simulink model "HANcoder_E407_DYS_MP"  (R2018b)
settings: Solver=FixedStepDiscrete  StartTime=0.0  StopTime=1  FixedStep=0.01  RelTol=1e-3
PreLoadFcn:
  | librarySetup
  | eval([bdroot,'_startup']) %Calling [modelName]_startup.m
values from neighbouring files (symbols this model uses):
  basic_cycle_duration_bc0 = TM_Reset_Board   + COMP_duration    (= 212)    [HANcoder_E407_DYS_MP_startup.m]
  basic_cycle_duration_bc1 = basic_cycle_duration_bc0    (= 212)    [HANcoder_E407_DYS_MP_startup.m]
  comm_delay_estimation1 = round(comm_delay_measured1*hardware_granularity/frequency_IRQ)    [HANcoder_E407_DYS_MP_startup.m]
  comm_delay_estimation2 = round(comm_delay_measured2*hardware_granularity/frequency_IRQ)    [HANcoder_E407_DYS_MP_startup.m]
  COMM_Phase1 = Simulink.Parameter    [HANcoder_E407_DYS_MP_startup.m]
  COMM_Phase2 = Simulink.Parameter    [HANcoder_E407_DYS_MP_startup.m]
  frequency_IRQ = 500    [HANcoder_E407_DYS_MP_startup.m]
  HantuneAngleSp = Simulink.Parameter    [HANcoder_E407_DYS_MP_startup.m]
  idle_time_init = basic_cycle_duration_bc0 + basic_cycle_duration_bc1    (= 424)    [HANcoder_E407_DYS_MP_startup.m]
  matrix_rows = 2    [HANcoder_E407_DYS_MP_startup.m]
  positionD = Simulink.Parameter    [HANcoder_E407_DYS_MP_startup.m]
  positionI = Simulink.Parameter    [HANcoder_E407_DYS_MP_startup.m]
  positionP = Simulink.Parameter    [HANcoder_E407_DYS_MP_startup.m]
undefined symbols (not defined in the file or in its folder): A1, CON2, CON4, D13, Dposition, Iposition, Pposition
libraries: HANcoder_STM32_Target x33, dspswit3 x16, simulink x2, simulink_extras x2, dspstat3 x1
(part 3 of 10)

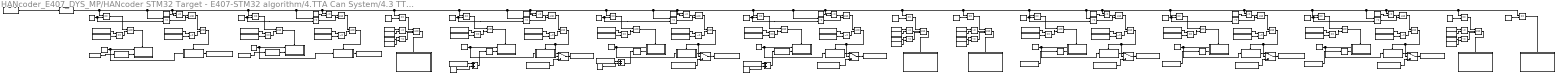
== system HANcoder_E407_DYS_MP/HANcoder STM32 Target - E407-STM32 algorithm/4.TTA Can System/4.3 TTA System/4.3.3 Matrix Cycle Manager/4.3.3.1 Controller Matrix Cycle Truck Boards 1 2 and 3/4.3.3.1.2 controller basic cycle 0.2 ==
  note: 4.3.3.1.2.1 Send Trailer Input angle 1
  note: 4.3.3.1.2.2 Receive Trailer Input angle 1
  note: 4.3.3.1.2.3 Send Trailer Input angle 2
  note: 4.3.3.1.2.4 Receive Trailer Input angle 2
  note: 4.3.3.1.2.6 Send Calc Steering Angle Board 1
  note: 4.3.3.1.2.7 Receive Calc Steering Angle Board 1
  note: 4.3.3.1.2.5 Calculate Articulation angle
  note: 4.3.3.1.2.8 Send Calc Steering Angle Board 2
  note: 4.3.3.1.2.9 Receive Calc Steering Angle Board 2
  note: 4.3.3.1.2.11 Receive Calc Steering Angle Board 3
  note: 4.3.3.1.2.10 Send Calc Steering Angle Board 3
  note: 4.3.3.1.2.12 Validate Articulation angle
  note: 4.3.3.1.2.13 Validated Angle to PWM
  note: 4.3.3.1.2.21 Check if Current id is equal to ID during initialization
  note: 4.3.3.1.2.14 Send Calc Encoder Value Board 1
  note: 4.3.3.1.2.15 Receive Calc Encoder Value Board 1
  note: 4.3.3.1.2.16 Send Calc Encoder Value Board 2
  note: 4.3.3.1.2.17 Receive Calc Encoder Value Board 2
  note: 4.3.3.1.2.19 Receive Calc Encoder Value Board 2
  note: 4.3.3.1.2.18 Send Calc Encoder Value Board 2
  note: 4.3.3.1.2.20 Check If Masters current encoder value is valid
  AND{1..6,8..16,19..27} (24 alike) : Logic  IconShape=distinctive  AllPortsSameDT=off  OutDataTypeStr=boolean
  AND{7,17..18,28} (4 alike) : Logic  Inputs=3  IconShape=distinctive  AllPortsSameDT=off  OutDataTypeStr=boolean
  Add : Sum
  Add1 : Sum
  Add2 : Sum
  Constant1 : Constant  Value=100
  Constant10 : Constant  Value=4
  Constant11 : Constant  Value=9  OutDataTypeStr=uint32
  Constant{12,17,47,50} (4 alike) : Constant  Value=2
  Constant13 : Constant  Value=95
  Constant14 : Constant  Value=94
  Constant15 : Constant  Value=99
  Constant16 : Constant  Value=8  OutDataTypeStr=uint32
  Constant18 : Constant  Value=105
  Constant19 : Constant  Value=109
  Constant{2,20..21,30,32,41,44,55} (8 alike) : Constant
  Constant22 : Constant  Value=5
  Constant23 : Constant  Value=4
  Constant{5,24..25,31,33,51,53,56} (8 alike) : Constant  Value=3
  Constant26 : Constant  Value=6  OutDataTypeStr=uint32
  Constant27 : Constant  Value=115
  Constant28 : Constant  Value=119
  Constant29 : Constant  Value=120
  Constant3 : Constant  Value=10  OutDataTypeStr=uint32
  Constant34 : Constant  Value=121
  Constant35 : Constant  Value=5  OutDataTypeStr=uint32
  Constant{8,36,38..39} (4 alike) : Constant  Value=90
  Constant37 : Constant  Value=138
  Constant4 : Constant  Value=7  OutDataTypeStr=uint32
  Constant40 : Constant  Value=122
  Constant42 : Constant  Value=3  OutDataTypeStr=uint32
  Constant43 : Constant  Value=126
  Constant45 : Constant  Value=4  OutDataTypeStr=uint32
  Constant46 : Constant  Value=127
  Constant48 : Constant  Value=132
  Constant49 : Constant  Value=131
  Constant52 : Constant  Value=136
  Constant54 : Constant  Value=137
  Constant6 : Constant  Value=110
  Constant7 : Constant  Value=114
  Constant9 : Constant  Value=5
  Data Store Read{,1..3,5..7,9,13..14,16..21,26,28,30,32,34,36..38} (24 alike) : DataStoreRead  DataStoreName=Board_ID
  Data Store Read10 : DataStoreRead  DataStoreName=Votes_Angle  DataStoreElements=Votes_Angle.First_Board
  Data Store Read11 : DataStoreRead  DataStoreName=Votes_Angle  DataStoreElements=Votes_Angle.Second_Board
  Data Store Read12 : DataStoreRead  DataStoreName=CalcSteeringAngle
  Data Store Read15 : DataStoreRead  DataStoreName=CalcSteeringAngle
  Data Store Read22 : DataStoreRead  DataStoreName=Votes_Angle  DataStoreElements=Votes_Angle.Third_Board
  Data Store Read23 : DataStoreRead  DataStoreName=PotAngle
  Data Store Read24 : DataStoreRead  DataStoreName=PotAngle
  Data Store Read25 : DataStoreRead  DataStoreName=EncoderValue
  Data Store Read27 : DataStoreRead  DataStoreName=Votes_Encoder  DataStoreElements=Votes_Encoder.First_Board
  Data Store Read29 : DataStoreRead  DataStoreName=EncoderValue
  Data Store Read31 : DataStoreRead  DataStoreName=Votes_Encoder  DataStoreElements=Votes_Encoder.Second_Board
  Data Store Read33 : DataStoreRead  DataStoreName=EncoderValue
  Data Store Read35 : DataStoreRead  DataStoreName=Votes_Encoder  DataStoreElements=Votes_Encoder.Third_Board
  Data Store Read4 : DataStoreRead  DataStoreName=CalcSteeringAngle
  Data Store Read8 : DataStoreRead  DataStoreName=Local_Ticks
  Data Store Write : DataStoreWrite  DataStoreName=InputAngle1
  Data Store Write1 : DataStoreWrite  DataStoreName=InputAngle2
  Data Store Write2 : DataStoreWrite  DataStoreName=Votes_Angle  DataStoreElements=Votes_Angle.First_Board
  Data Store Write3 : DataStoreWrite  DataStoreName=Votes_Angle  DataStoreElements=Votes_Angle.Second_Board
  Data Store Write4 : DataStoreWrite  DataStoreName=Votes_Angle  DataStoreElements=Votes_Angle.Third_Board
  Data Store Write6 : DataStoreWrite  DataStoreName=Votes_Encoder  DataStoreElements=Votes_Encoder.First_Board
  Data Store Write7 : DataStoreWrite  DataStoreName=Votes_Encoder  DataStoreElements=Votes_Encoder.Second_Board
  Data Store Write8 : DataStoreWrite  DataStoreName=Votes_Encoder  DataStoreElements=Votes_Encoder.Third_Board
  Data Type Conversion{1..2,4..9} (8 alike) : DataTypeConversion  OutDataTypeStr=uint8
  Data Type Conversion3 : DataTypeConversion  OutDataTypeStr=double
  Equal{1,13,15,23} (4 alike) : RelationalOperator  OutDataTypeStr=boolean  RndMeth=Simplest
  Equal{5..7,10..11,17,19,21} (8 alike) : RelationalOperator  Operator===  OutDataTypeStr=boolean  RndMeth=Simplest
  Equal{2..4,9,12,18,20,22} (8 alike) : RelationalOperator  Operator=~=  OutDataTypeStr=boolean  RndMeth=Simplest
  Equal{8,14,16,24} (4 alike) : RelationalOperator  Operator=<=  OutDataTypeStr=boolean  RndMeth=Simplest
  GreaterThanOrEqual{1..2,4,6,10,15,17..20,23,26,29} (13 alike) : RelationalOperator  Operator===  OutDataTypeStr=boolean  RndMeth=Simplest
  GreaterThanOrEqual{3,5,7,11,16,21,24,27} (8 alike) : RelationalOperator  OutDataTypeStr=boolean  RndMeth=Simplest
  GreaterThanOrEqual{8..9,12..14,22,25,28} (8 alike) : RelationalOperator  Operator=<=  OutDataTypeStr=boolean  RndMeth=Simplest
  If Action Subsystem : Subsystem  TreatAsAtomicUnit=on
  If Action Subsystem1 : Subsystem  TreatAsAtomicUnit=on
  If Action Subsystem2 : Subsystem  TreatAsAtomicUnit=on
  If Action Subsystem3 : Subsystem  TreatAsAtomicUnit=on
  If Action Subsystem4 : Subsystem  TreatAsAtomicUnit=on
  Receive Trailer 1 board 4 input angel : Subsystem
  Receive Trailer 2 board 5 input angel : Subsystem
  Receive Truck 1 Board 1 Calc Steering Angle : Subsystem
  Receive Truck 1 Board 1 Calc Steering Angle1 : Subsystem
  Receive Truck 1 Board 1 Calc Steering Angle2 : Subsystem
  Receive Truck 1 Board 1 Calc Steering Angle3 : Subsystem
  Receive Truck 2 Board 2 Calc Steering Angle : Subsystem
  Receive Truck 3 Board 3 Calc Steering Angle : Subsystem
  Send can message : Subsystem  TreatAsAtomicUnit=on
  Send can message1 : Subsystem  TreatAsAtomicUnit=on
  Send can message2 : Subsystem  TreatAsAtomicUnit=on
  Send can message3 : Subsystem  TreatAsAtomicUnit=on
  Send can message4 : Subsystem  TreatAsAtomicUnit=on
  Send can message5 : Subsystem  TreatAsAtomicUnit=on
  Send can message6 : Subsystem  TreatAsAtomicUnit=on
  Send can message7 : Subsystem  TreatAsAtomicUnit=on
  Switch{,1..5} (6 alike) : Switch  Criteria=u2 > Threshold
  wires:
  Data Store Read8/1 -> Data Type Conversion3/1
  Constant8/1 -> GreaterThanOrEqual5/2, GreaterThanOrEqual4/2
  Equal2/1 -> AND9/2
  Data Store Read/1 -> Equal2/1
  Constant10/1 -> Equal2/2
  AND9/1 -> Receive Trailer 1 board 4 input angel/Enable
  Constant3/1 -> Receive Trailer 1 board 4 input angel/1(Input), Send can message/1(Can_ID)
  AND6/1 -> Receive Trailer 2 board 5 input angel/Enable
  Constant13/1 -> GreaterThanOrEqual7/2, GreaterThanOrEqual6/2
  Data Store Read2/1 -> Equal3/1
  Equal3/1 -> AND6/2
  Constant9/1 -> Equal3/2
  Constant11/1 -> Receive Trailer 2 board 5 input angel/1(Input), Send can message1/1(Can_ID)
  Constant14/1 -> GreaterThanOrEqual8/2
  GreaterThanOrEqual8/1 -> AND3/1
  GreaterThanOrEqual5/1 -> AND3/2
  AND3/1 -> AND9/1
  Receive Trailer 1 board 4 input angel/1(Angle) -> Data Store Write/1
  Constant15/1 -> GreaterThanOrEqual9/2
  GreaterThanOrEqual9/1 -> AND4/1
  GreaterThanOrEqual7/1 -> AND4/2
  AND4/1 -> AND6/1
  Receive Trailer 2 board 5 input angel/1(Angle) -> Data Store Write1/1
  Constant18/1 -> GreaterThanOrEqual11/2, GreaterThanOrEqual10/2
  GreaterThanOrEqual11/1 -> AND5/2
  AND2/1 -> Switch/2, Receive Truck 1 Board 1 Calc Steering Angle/Enable
  Constant16/1 -> Receive Truck 1 Board 1 Calc Steering Angle/1(Input), Send can message2/1(Can_ID)
  Constant20/1 -> Equal4/2
  Equal4/1 -> AND2/2
  AND5/1 -> AND2/1
  GreaterThanOrEqual12/1 -> AND5/1
  Data Store Read5/1 -> Equal4/1
  Constant19/1 -> GreaterThanOrEqual12/2
  Equal5/1 -> AND1/2
  Constant21/1 -> Equal5/2
  Data Store Read6/1 -> Equal5/1
  AND1/1 -> Send can message2/Enable
  GreaterThanOrEqual10/1 -> AND1/1
  Equal6/1 -> AND8/2
  Constant22/1 -> Equal6/2
  Data Store Read7/1 -> Equal6/1
  GreaterThanOrEqual6/1 -> AND8/1
  AND8/1 -> Send can message1/Enable
  GreaterThanOrEqual4/1 -> AND10/1
  Data Store Read9/1 -> Equal7/1
  Constant23/1 -> Equal7/2
  Equal7/1 -> AND10/2
  AND10/1 -> Send can message/Enable
  Constant1/1 -> GreaterThanOrEqual1/2
  GreaterThanOrEqual1/1 -> AND7/1
  AND7/1 -> If Action Subsystem/Enable
  Data Store Read1/1 -> Equal1/1
  Constant2/1 -> Equal1/2
  Equal1/1 -> AND7/2
  Constant5/1 -> Equal8/2
  Data Store Read3/1 -> Equal8/1
  Equal8/1 -> AND7/3
  GreaterThanOrEqual3/1 -> AND13/2
  Data Store Read14/1 -> Equal10/1
  Constant7/1 -> GreaterThanOrEqual13/2
  GreaterThanOrEqual13/1 -> AND13/1
  Constant4/1 -> Receive Truck 2 Board 2 Calc Steering Angle/1(Input), Send can message3/1(Can_ID)
  Constant6/1 -> GreaterThanOrEqual3/2, GreaterThanOrEqual2/2
  Constant17/1 -> Equal10/2
  GreaterThanOrEqual2/1 -> AND11/1
  Equal10/1 -> AND11/2
  AND11/1 -> Send can message3/Enable
  Data Store Read13/1 -> Equal9/1
  Constant12/1 -> Equal9/2
  AND13/1 -> AND12/1
  Equal9/1 -> AND12/2
  GreaterThanOrEqual14/1 -> AND16/1
  Data Store Read17/1 -> Equal11/1
  GreaterThanOrEqual16/1 -> AND16/2
  Constant28/1 -> GreaterThanOrEqual14/2
  Equal12/1 -> AND15/2
  Equal11/1 -> AND14/2
  GreaterThanOrEqual15/1 -> AND14/1
  AND16/1 -> AND15/1
  Data Store Read16/1 -> Equal12/1
  AND14/1 -> Send can message4/Enable
  Constant27/1 -> GreaterThanOrEqual16/2, GreaterThanOrEqual15/2
  Constant25/1 -> Equal11/2
  Constant26/1 -> Receive Truck 3 Board 3 Calc Steering Angle/1(Input), Send can message4/1(Can_ID)
  Constant24/1 -> Equal12/2
  Data Store Read19/1 -> Equal14/1
  GreaterThanOrEqual17/1 -> AND17/1
  AND17/1 -> If Action Subsystem1/Enable
  Constant29/1 -> GreaterThanOrEqual17/2
  Constant30/1 -> Equal13/2
  Constant31/1 -> Equal14/2
  Data Store Read18/1 -> Equal13/1
  Equal14/1 -> AND17/3
  Equal13/1 -> AND17/2
  Data Store Read20/1 -> Equal15/1
  Equal16/1 -> AND18/3
  Equal15/1 -> AND18/2
  Constant32/1 -> Equal15/2
  Constant33/1 -> Equal16/2
  GreaterThanOrEqual18/1 -> AND18/1
  Data Store Read21/1 -> Equal16/1
  Constant34/1 -> GreaterThanOrEqual18/2
  AND18/1 -> If Action Subsystem2/Enable
  GreaterThanOrEqual19/1 -> If Action Subsystem3/Enable
  Constant37/1 -> GreaterThanOrEqual19/2
  Data Store Read24/1 -> Data Type Conversion2/1
  Data Type Conversion2/1 -> Send can message1/2(Can_Data)
  Data Type Conversion1/1 -> Send can message/2(Can_Data)
  Data Store Read23/1 -> Data Type Conversion1/1
  Data Type Conversion4/1 -> Send can message2/2(Can_Data)
  Data Type Conversion5/1 -> Send can message3/2(Can_Data)
  Data Type Conversion6/1 -> Send can message4/2(Can_Data)
  Data Store Read12/1 -> Add/1
  Constant36/1 -> Add/2
  Add/1 -> Data Type Conversion5/1
  Constant38/1 -> Add1/2
  Data Store Read15/1 -> Add1/1
  Add1/1 -> Data Type Conversion6/1
  Constant39/1 -> Add2/2
  Add2/1 -> Data Type Conversion4/1  "testtest"
  Data Store Read4/1 -> Add2/1  "test1"
  Switch/1 -> Data Store Write2/1
  Receive Truck 1 Board 1 Calc Steering Angle/1(Angle) -> Switch/1
  Data Store Read10/1 -> Switch/3
  AND12/1 -> Switch1/2, Receive Truck 2 Board 2 Calc Steering Angle/Enable
  Data Store Read11/1 -> Switch1/3
  Receive Truck 2 Board 2 Calc Steering Angle/1(Angle) -> Switch1/1
  Switch1/1 -> Data Store Write3/1
  Switch2/1 -> Data Store Write4/1
  AND15/1 -> Switch2/2, Receive Truck 3 Board 3 Calc Steering Angle/Enable
  Data Store Read22/1 -> Switch2/3
  Receive Truck 3 Board 3 Calc Steering Angle/1(Angle) -> Switch2/1
  Constant41/1 -> Equal17/2
  Data Store Read25/1 -> Data Type Conversion7/1
  Data Type Conversion7/1 -> Send can message5/2(Can_Data)
  Constant40/1 -> GreaterThanOrEqual21/2, GreaterThanOrEqual20/2
  Data Store Read26/1 -> Equal17/1
  Equal17/1 -> AND19/2
  GreaterThanOrEqual20/1 -> AND19/1
  AND19/1 -> Send can message5/Enable
  GreaterThanOrEqual21/1 -> AND21/2
  Constant43/1 -> GreaterThanOrEqual22/2
  Data Store Read28/1 -> Equal18/1
  AND21/1 -> AND20/1
  GreaterThanOrEqual22/1 -> AND21/1
  Constant35/1 -> Receive Truck 1 Board 1 Calc Steering Angle1/1(Input), Send can message5/1(Can_ID)
  Constant44/1 -> Equal18/2
  Receive Truck 1 Board 1 Calc Steering Angle1/1(Angle) -> Switch3/1
  AND20/1 -> Switch3/2, Receive Truck 1 Board 1 Calc Steering Angle1/Enable
  Data Store Read27/1 -> Switch3/3
  Switch3/1 -> Data Store Write6/1
  Equal18/1 -> AND20/2
  Switch4/1 -> Data Store Write7/1
  Data Store Read29/1 -> Data Type Conversion8/1
  AND23/1 -> Switch4/2, Receive Truck 1 Board 1 Calc Steering Angle2/Enable
  Equal20/1 -> AND23/2
  Receive Truck 1 Board 1 Calc Steering Angle2/1(Angle) -> Switch4/1
  Data Store Read31/1 -> Switch4/3
  GreaterThanOrEqual25/1 -> AND24/1
  Data Store Read32/1 -> Equal20/1
  AND24/1 -> AND23/1
  GreaterThanOrEqual24/1 -> AND24/2
  Constant50/1 -> Equal20/2
  AND22/1 -> Send can message6/Enable
  Constant49/1 -> GreaterThanOrEqual25/2
  Constant45/1 -> Receive Truck 1 Board 1 Calc Steering Angle2/1(Input), Send can message6/1(Can_ID)
  Equal19/1 -> AND22/2
  Data Store Read30/1 -> Equal19/1
  Data Type Conversion8/1 -> Send can message6/2(Can_Data)
  Constant46/1 -> GreaterThanOrEqual24/2, GreaterThanOrEqual23/2
  GreaterThanOrEqual23/1 -> AND22/1
  Constant47/1 -> Equal19/2
  Constant51/1 -> Equal21/2
  Constant52/1 -> GreaterThanOrEqual28/2
  AND25/1 -> Send can message7/Enable
  Constant53/1 -> Equal22/2
  GreaterThanOrEqual27/1 -> AND27/2
  AND27/1 -> AND26/1
  GreaterThanOrEqual28/1 -> AND27/1
  Data Store Read36/1 -> Equal22/1
  Receive Truck 1 Board 1 Calc Steering Angle3/1(Angle) -> Switch5/1
  Equal22/1 -> AND26/2
  AND26/1 -> Switch5/2, Receive Truck 1 Board 1 Calc Steering Angle3/Enable
  Switch5/1 -> Data Store Write8/1
  Data Store Read35/1 -> Switch5/3
  Constant48/1 -> GreaterThanOrEqual27/2, GreaterThanOrEqual26/2
  Data Store Read34/1 -> Equal21/1
  Data Type Conversion9/1 -> Send can message7/2(Can_Data)
  Equal21/1 -> AND25/2
  Constant42/1 -> Receive Truck 1 Board 1 Calc Steering Angle3/1(Input), Send can message7/1(Can_ID)
  Data Store Read33/1 -> Data Type Conversion9/1
  GreaterThanOrEqual26/1 -> AND25/1
  Data Type Conversion3/1 -> GreaterThanOrEqual8/1, GreaterThanOrEqual11/1, GreaterThanOrEqual3/1, GreaterThanOrEqual21/1, GreaterThanOrEqual22/1, GreaterThanOrEqual23/1, GreaterThanOrEqual25/1, GreaterThanOrEqual26/1, GreaterThanOrEqual27/1, GreaterThanOrEqual28/1, GreaterThanOrEqual29/1, GreaterThanOrEqual19/1, GreaterThanOrEqual20/1, GreaterThanOrEqual18/1, GreaterThanOrEqual17/1, GreaterThanOrEqual14/1, GreaterThanOrEqual16/1, GreaterThanOrEqual15/1, GreaterThanOrEqual13/1, GreaterThanOrEqual2/1, GreaterThanOrEqual12/1, GreaterThanOrEqual10/1, GreaterThanOrEqual1/1, GreaterThanOrEqual9/1, GreaterThanOrEqual7/1, GreaterThanOrEqual6/1, GreaterThanOrEqual5/1, GreaterThanOrEqual4/1
  Constant56/1 -> Equal24/2
  AND28/1 -> If Action Subsystem4/Enable
  Data Store Read37/1 -> Equal23/1
  Constant55/1 -> Equal23/2
  Equal24/1 -> AND28/3
  Equal23/1 -> AND28/2
  GreaterThanOrEqual29/1 -> AND28/1
  Data Store Read38/1 -> Equal24/1
  Constant54/1 -> GreaterThanOrEqual29/2

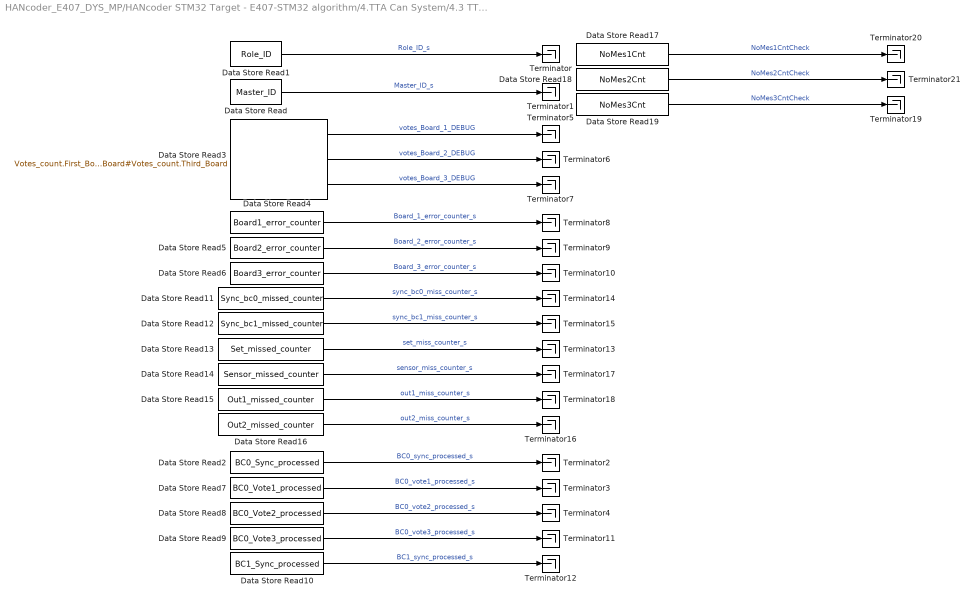
== system HANcoder_E407_DYS_MP/HANcoder STM32 Target - E407-STM32 algorithm/4.TTA Can System/4.3 TTA System/4.3.3 Matrix Cycle Manager/4.3.3.1 Controller Matrix Cycle Truck Boards 1 2 and 3/Matrix_Cycle_Observation_DEBUG ==
  Data Store Read : DataStoreRead  DataStoreName=Master_ID
  Data Store Read1 : DataStoreRead  DataStoreName=Role_ID
  Data Store Read10 : DataStoreRead  DataStoreName=BC1_Sync_processed
  Data Store Read11 : DataStoreRead  DataStoreName=Sync_bc0_missed_counter
  Data Store Read12 : DataStoreRead  DataStoreName=Sync_bc1_missed_counter
  Data Store Read13 : DataStoreRead  DataStoreName=Set_missed_counter
  Data Store Read14 : DataStoreRead  DataStoreName=Sensor_missed_counter
  Data Store Read15 : DataStoreRead  DataStoreName=Out1_missed_counter
  Data Store Read16 : DataStoreRead  DataStoreName=Out2_missed_counter
  Data Store Read17 : DataStoreRead  DataStoreName=NoMes1Cnt
  Data Store Read18 : DataStoreRead  DataStoreName=NoMes2Cnt
  Data Store Read19 : DataStoreRead  DataStoreName=NoMes3Cnt
  Data Store Read2 : DataStoreRead  DataStoreName=BC0_Sync_processed
  Data Store Read3 : DataStoreRead  DataStoreName=Votes_count  DataStoreElements=Votes_count.First_Board#Votes_count.Second_Board#Votes_count.Third_Board
  Data Store Read4 : DataStoreRead  DataStoreName=Board1_error_counter
  Data Store Read5 : DataStoreRead  DataStoreName=Board2_error_counter
  Data Store Read6 : DataStoreRead  DataStoreName=Board3_error_counter
  Data Store Read7 : DataStoreRead  DataStoreName=BC0_Vote1_processed
  Data Store Read8 : DataStoreRead  DataStoreName=BC0_Vote2_processed
  Data Store Read9 : DataStoreRead  DataStoreName=BC0_Vote3_processed
  Terminator{,1..21} (22 alike) : Terminator
  wires:
  Data Store Read/1 -> Terminator1/1  "Master_ID_s"
  Data Store Read3/1 -> Terminator5/1  "votes_Board_1_DEBUG"
  Data Store Read3/2 -> Terminator6/1  "votes_Board_2_DEBUG"
  Data Store Read3/3 -> Terminator7/1  "votes_Board_3_DEBUG"
  Data Store Read4/1 -> Terminator8/1  "Board_1_error_counter_s"
  Data Store Read5/1 -> Terminator9/1  "Board_2_error_counter_s"
  Data Store Read6/1 -> Terminator10/1  "Board_3_error_counter_s"
  Data Store Read2/1 -> Terminator2/1  "BC0_sync_processed_s"
  Data Store Read7/1 -> Terminator3/1  "BC0_vote1_processed_s"
  Data Store Read8/1 -> Terminator4/1  "BC0_vote2_processed_s"
  Data Store Read9/1 -> Terminator11/1  "BC0_vote3_processed_s"
  Data Store Read10/1 -> Terminator12/1  "BC1_sync_processed_s"
  Data Store Read1/1 -> Terminator/1  "Role_ID_s"
  Data Store Read11/1 -> Terminator14/1  "sync_bc0_miss_counter_s"
  Data Store Read12/1 -> Terminator15/1  "sync_bc1_miss_counter_s"
  Data Store Read13/1 -> Terminator13/1  "set_miss_counter_s"
  Data Store Read14/1 -> Terminator17/1  "sensor_miss_counter_s"
  Data Store Read15/1 -> Terminator18/1  "out1_miss_counter_s"
  Data Store Read16/1 -> Terminator16/1  "out2_miss_counter_s"
  Data Store Read17/1 -> Terminator20/1  "NoMes1CntCheck"
  Data Store Read18/1 -> Terminator21/1  "NoMes2CntCheck"
  Data Store Read19/1 -> Terminator19/1  "NoMes3CntCheck"

== system HANcoder_E407_DYS_MP/HANcoder STM32 Target - E407-STM32 algorithm/4.TTA Can System/4.3 TTA System/4.3.3 Matrix Cycle Manager/4.3.3.1 Controller Matrix Cycle Truck Boards 1 2 and 3/msg_count_DEBUG observer ==
  Data Store Read24 : DataStoreRead  DataStoreName=msg_count_DEBUG
  Terminator : Terminator
  wires:
  Data Store Read24/1 -> Terminator/1  "msg_count_DEBUG_s"

== system HANcoder_E407_DYS_MP/HANcoder STM32 Target - E407-STM32 algorithm/4.TTA Can System/4.3 TTA System/4.3.3 Matrix Cycle Manager/4.3.3.2 Controller Matrix Cycle_Board 4 and 5/controller basic cycle 0 ==
  note: Receving Time Window
  note: Receving Time Window
  AND : Logic  IconShape=distinctive  AllPortsSameDT=off  OutDataTypeStr=boolean
  AND1 : Logic  IconShape=distinctive  AllPortsSameDT=off  OutDataTypeStr=boolean
  AND2 : Logic  IconShape=distinctive  AllPortsSameDT=off  OutDataTypeStr=boolean
  Constant : Constant  Value=25
  Constant5 : Constant  Value=5
  Constant6 : Constant  Value=60
  Constant7 : Constant  Value=61
  Counter1 : dspswit3/Counter  Direction=Up  CountEvent=Rising edge  CounterSize=User defined  MaxCount=255  InitialCount=0  Output=Count and Hit  HitValue=32  ResetInput=on  SamplesPerFrame=1  Ts=1  CntDtype=double  HitDtype=Logical
  Counter3 : dspswit3/Counter  Direction=Up  CountEvent=Rising edge  CounterSize=User defined  MaxCount=255  InitialCount=0  Output=Count and Hit  HitValue=32  ResetInput=on  SamplesPerFrame=1  Ts=1  CntDtype=double  HitDtype=Logical
  Data Store Memory3 : DataStoreMemory  DataStoreName=SyncMesRec  ReadBeforeWriteMsg=warning  WriteAfterWriteMsg=warning  WriteAfterReadMsg=warning  ShowAdditionalParam=off  OutMin=0  OutMax=255  OutDataTypeStr=uint8
  Data Store Read3 : DataStoreRead  Priority=10  DataStoreName=Role_ID
  Data Store Read4 : DataStoreRead  DataStoreName=SyncMesRec
  Data Store Read8 : DataStoreRead  DataStoreName=Local_Ticks
  Data Type Conversion3 : DataTypeConversion  OutDataTypeStr=double
  Desync calculation : Subsystem  Priority=10
  GreaterThanOrEqual : RelationalOperator  Operator=>  OutDataTypeStr=boolean  RndMeth=Simplest
  GreaterThanOrEqual1 : RelationalOperator  Operator=<=  OutDataTypeStr=boolean  RndMeth=Simplest
  GreaterThanOrEqual2 : RelationalOperator  Operator=>  OutDataTypeStr=boolean  RndMeth=Simplest
  GreaterThanOrEqual3 : RelationalOperator  Operator=<=  OutDataTypeStr=boolean  RndMeth=Simplest
  If Action Subsystem : Subsystem  TreatAsAtomicUnit=on
  OR : Logic  Operator=OR  IconShape=distinctive  AllPortsSameDT=off  OutDataTypeStr=boolean
  "Receive Timer can master message " : Subsystem
  Terminator1 : Terminator
  Terminator4 : Terminator
  wires:
  Data Store Read8/1 -> Data Type Conversion3/1
  Data Type Conversion3/1 -> GreaterThanOrEqual/1, GreaterThanOrEqual1/1, GreaterThanOrEqual2/1, GreaterThanOrEqual3/1
  Data Store Read3/1 -> "Receive Timer can master message "/1(Sender Id)
  Constant/1 -> Desync calculation/1(TM_COMM)
  "Receive Timer can master message "/2(Can1Rec) -> OR/1, Desync calculation/2(New_msg_CAN1)
  "Receive Timer can master message "/4(Can2Rec) -> OR/2
  OR/1 -> Counter1/1, Desync calculation/Enable
  Constant5/1 -> GreaterThanOrEqual/2
  GreaterThanOrEqual/1 -> AND/2
  Constant6/1 -> GreaterThanOrEqual2/2, GreaterThanOrEqual1/2
  GreaterThanOrEqual1/1 -> AND/1
  Constant7/1 -> GreaterThanOrEqual3/2
  GreaterThanOrEqual3/1 -> AND1/1
  GreaterThanOrEqual2/1 -> AND1/2
  AND2/1 -> If Action Subsystem/Enable
  Counter1/1 -> Terminator1/1
  Counter3/1 -> Terminator4/1
  AND/1 -> Counter3/1, "Receive Timer can master message "/Enable
  AND1/1 -> AND2/1
  Data Store Read4/1 -> AND2/2

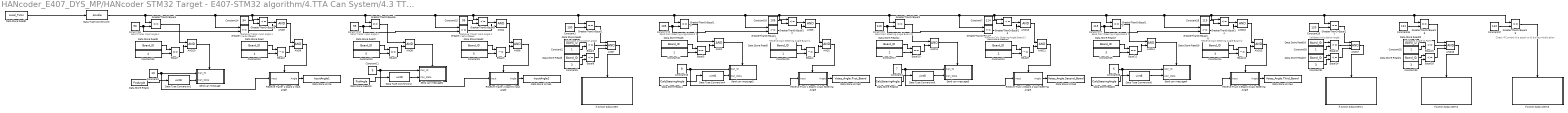
== system HANcoder_E407_DYS_MP/HANcoder STM32 Target - E407-STM32 algorithm/4.TTA Can System/4.3 TTA System/4.3.3 Matrix Cycle Manager/4.3.3.2 Controller Matrix Cycle_Board 4 and 5/controller basic cycle 0.2 ==
  note: Send Trailer Input angle 1
  note: Receive Trailer Input angle 1
  note: Send Trailer Input angle 2
  note: Receive Trailer Input angle 2
  note: Send Calc Steering Angle Board 1
  note: Receive Calc Steering Angle Board 1
  note: Calculate Articulation angle
  note: Send Calc Steering Angle Board 2
  note: Receive Calc Steering Angle Board 2
  note: Receive Calc Steering Angle Board 2
  note: Send Calc Steering Angle Board 2
  note: Validate Articulation angle
  note: Validated Angle to PWM
  note: Check if Current id is equal to ID during initialization
  AND{1..6,8..16} (15 alike) : Logic  IconShape=distinctive  AllPortsSameDT=off  OutDataTypeStr=boolean
  AND17 : Logic  Inputs=3  IconShape=distinctive  AllPortsSameDT=off  OutDataTypeStr=boolean
  AND18 : Logic  Inputs=3  IconShape=distinctive  AllPortsSameDT=off  OutDataTypeStr=boolean
  AND7 : Logic  Inputs=3  IconShape=distinctive  AllPortsSameDT=off  OutDataTypeStr=boolean
  Constant1 : Constant  Value=100
  Constant10 : Constant  Value=4
  Constant11 : Constant  Value=9  OutDataTypeStr=uint32
  Constant12 : Constant  Value=2
  Constant13 : Constant  Value=95
  Constant14 : Constant  Value=94
  Constant15 : Constant  Value=99
  Constant16 : Constant  Value=8  OutDataTypeStr=uint32
  Constant17 : Constant  Value=2
  Constant18 : Constant  Value=105
  Constant19 : Constant  Value=109
  Constant{2,20..21,30,32} (5 alike) : Constant
  Constant22 : Constant  Value=5
  Constant23 : Constant  Value=4
  Constant{5,24..25,31,33} (5 alike) : Constant  Value=3
  Constant26 : Constant  Value=6  OutDataTypeStr=uint32
  Constant27 : Constant  Value=115
  Constant28 : Constant  Value=119
  Constant29 : Constant  Value=120
  Constant3 : Constant  Value=10  OutDataTypeStr=uint32
  Constant34 : Constant  Value=121
  Constant37 : Constant  Value=122
  Constant4 : Constant  Value=7  OutDataTypeStr=uint32
  Constant6 : Constant  Value=110
  Constant7 : Constant  Value=114
  Constant8 : Constant  Value=90
  Constant9 : Constant  Value=5
  Data Store Read{,1..3,5..7,9,13..14,16..21} (16 alike) : DataStoreRead  DataStoreName=Board_ID
  Data Store Read10 : DataStoreRead  DataStoreName=PotAngle
  Data Store Read11 : DataStoreRead  DataStoreName=CalcSteeringAngle
  Data Store Read12 : DataStoreRead  DataStoreName=CalcSteeringAngle
  Data Store Read15 : DataStoreRead  DataStoreName=CalcSteeringAngle
  Data Store Read4 : DataStoreRead  DataStoreName=PotAngle
  Data Store Read8 : DataStoreRead  DataStoreName=Local_Ticks
  Data Store Write : DataStoreWrite  DataStoreName=InputAngle1
  Data Store Write1 : DataStoreWrite  DataStoreName=InputAngle2
  Data Store Write2 : DataStoreWrite  DataStoreName=Votes_Angle  DataStoreElements=Votes_Angle.First_Board
  Data Store Write3 : DataStoreWrite  DataStoreName=Votes_Angle  DataStoreElements=Votes_Angle.Second_Board
  Data Store Write4 : DataStoreWrite  DataStoreName=Votes_Angle  DataStoreElements=Votes_Angle.Third_Board
  Data Type Conversion{1..2,4..6} (5 alike) : DataTypeConversion  OutDataTypeStr=uint8
  Data Type Conversion3 : DataTypeConversion  OutDataTypeStr=double
  Equal1 : RelationalOperator  OutDataTypeStr=boolean  RndMeth=Simplest
  Equal{5..7,10..11} (5 alike) : RelationalOperator  Operator===  OutDataTypeStr=boolean  RndMeth=Simplest
  Equal{2..4,9,12} (5 alike) : RelationalOperator  Operator=~=  OutDataTypeStr=boolean  RndMeth=Simplest
  Equal13 : RelationalOperator  OutDataTypeStr=boolean  RndMeth=Simplest
  Equal14 : RelationalOperator  Operator=<=  OutDataTypeStr=boolean  RndMeth=Simplest
  Equal15 : RelationalOperator  OutDataTypeStr=boolean  RndMeth=Simplest
  Equal16 : RelationalOperator  Operator=<=  OutDataTypeStr=boolean  RndMeth=Simplest
  Equal8 : RelationalOperator  Operator=<=  OutDataTypeStr=boolean  RndMeth=Simplest
  GreaterThanOrEqual{1..2,4,6,10,15,17..19} (9 alike) : RelationalOperator  Operator===  OutDataTypeStr=boolean  RndMeth=Simplest
  GreaterThanOrEqual{3,5,7,11,16} (5 alike) : RelationalOperator  OutDataTypeStr=boolean  RndMeth=Simplest
  GreaterThanOrEqual{8..9,12..14} (5 alike) : RelationalOperator  Operator=<=  OutDataTypeStr=boolean  RndMeth=Simplest
  If Action Subsystem : Subsystem  TreatAsAtomicUnit=on
  If Action Subsystem1 : Subsystem  TreatAsAtomicUnit=on
  If Action Subsystem2 : Subsystem  TreatAsAtomicUnit=on
  If Action Subsystem3 : Subsystem  TreatAsAtomicUnit=on
  Receive Trailer 1 board 4 input angel : Subsystem
  Receive Trailer 2 board 5 input angel : Subsystem
  Receive Truck 1 Board 1 Calc Steering Angle : Subsystem
  Receive Truck 2 Board 2 Calc Steering Angle : Subsystem
  Receive Truck 3 Board 3 Calc Steering Angle : Subsystem
  Send can message : Subsystem  TreatAsAtomicUnit=on
  Send can message1 : Subsystem  TreatAsAtomicUnit=on
  Send can message2 : Subsystem  TreatAsAtomicUnit=on
  Send can message3 : Subsystem  TreatAsAtomicUnit=on
  Send can message4 : Subsystem  TreatAsAtomicUnit=on
  wires:
  Data Store Read8/1 -> Data Type Conversion3/1
  Constant8/1 -> GreaterThanOrEqual5/2, GreaterThanOrEqual4/2
  Equal2/1 -> AND9/2
  Data Store Read/1 -> Equal2/1
  Constant10/1 -> Equal2/2
  AND9/1 -> Receive Trailer 1 board 4 input angel/Enable
  Constant3/1 -> Receive Trailer 1 board 4 input angel/1(Input), Send can message/1(Can_ID)
  AND6/1 -> Receive Trailer 2 board 5 input angel/Enable
  Constant13/1 -> GreaterThanOrEqual7/2, GreaterThanOrEqual6/2
  Data Store Read2/1 -> Equal3/1
  Equal3/1 -> AND6/2
  Constant9/1 -> Equal3/2
  Constant11/1 -> Receive Trailer 2 board 5 input angel/1(Input), Send can message1/1(Can_ID)
  Constant14/1 -> GreaterThanOrEqual8/2
  GreaterThanOrEqual8/1 -> AND3/1
  GreaterThanOrEqual5/1 -> AND3/2
  AND3/1 -> AND9/1
  Receive Trailer 1 board 4 input angel/1(Angle) -> Data Store Write/1
  Constant15/1 -> GreaterThanOrEqual9/2
  GreaterThanOrEqual9/1 -> AND4/1
  GreaterThanOrEqual7/1 -> AND4/2
  AND4/1 -> AND6/1
  Receive Trailer 2 board 5 input angel/1(Angle) -> Data Store Write1/1
  Constant18/1 -> GreaterThanOrEqual11/2, GreaterThanOrEqual10/2
  GreaterThanOrEqual11/1 -> AND5/2
  AND2/1 -> Receive Truck 1 Board 1 Calc Steering Angle/Enable
  Receive Truck 1 Board 1 Calc Steering Angle/1(Angle) -> Data Store Write2/1
  Constant16/1 -> Receive Truck 1 Board 1 Calc Steering Angle/1(Input), Send can message2/1(Can_ID)
  Constant20/1 -> Equal4/2
  Equal4/1 -> AND2/2
  AND5/1 -> AND2/1
  GreaterThanOrEqual12/1 -> AND5/1
  Data Store Read5/1 -> Equal4/1
  Constant19/1 -> GreaterThanOrEqual12/2
  Equal5/1 -> AND1/2
  Constant21/1 -> Equal5/2
  Data Store Read6/1 -> Equal5/1
  AND1/1 -> Send can message2/Enable
  GreaterThanOrEqual10/1 -> AND1/1
  Equal6/1 -> AND8/2
  Constant22/1 -> Equal6/2
  Data Store Read7/1 -> Equal6/1
  GreaterThanOrEqual6/1 -> AND8/1
  AND8/1 -> Send can message1/Enable
  GreaterThanOrEqual4/1 -> AND10/1
  Data Store Read9/1 -> Equal7/1
  Constant23/1 -> Equal7/2
  Equal7/1 -> AND10/2
  AND10/1 -> Send can message/Enable
  Constant1/1 -> GreaterThanOrEqual1/2
  GreaterThanOrEqual1/1 -> AND7/1
  AND7/1 -> If Action Subsystem/Enable
  Data Store Read1/1 -> Equal1/1
  Constant2/1 -> Equal1/2
  Equal1/1 -> AND7/2
  Constant5/1 -> Equal8/2
  Data Store Read3/1 -> Equal8/1
  Equal8/1 -> AND7/3
  Receive Truck 2 Board 2 Calc Steering Angle/1(Angle) -> Data Store Write3/1
  GreaterThanOrEqual3/1 -> AND13/2
  Data Store Read14/1 -> Equal10/1
  Constant7/1 -> GreaterThanOrEqual13/2
  GreaterThanOrEqual13/1 -> AND13/1
  Constant4/1 -> Receive Truck 2 Board 2 Calc Steering Angle/1(Input), Send can message3/1(Can_ID)
  Constant6/1 -> GreaterThanOrEqual3/2, GreaterThanOrEqual2/2
  AND12/1 -> Receive Truck 2 Board 2 Calc Steering Angle/Enable
  Constant17/1 -> Equal10/2
  GreaterThanOrEqual2/1 -> AND11/1
  Equal10/1 -> AND11/2
  AND11/1 -> Send can message3/Enable
  Data Store Read13/1 -> Equal9/1
  Constant12/1 -> Equal9/2
  AND13/1 -> AND12/1
  Equal9/1 -> AND12/2
  GreaterThanOrEqual14/1 -> AND16/1
  Receive Truck 3 Board 3 Calc Steering Angle/1(Angle) -> Data Store Write4/1
  Data Store Read17/1 -> Equal11/1
  GreaterThanOrEqual16/1 -> AND16/2
  Constant28/1 -> GreaterThanOrEqual14/2
  Equal12/1 -> AND15/2
  Equal11/1 -> AND14/2
  GreaterThanOrEqual15/1 -> AND14/1
  AND16/1 -> AND15/1
  Data Store Read16/1 -> Equal12/1
  AND14/1 -> Send can message4/Enable
  Constant27/1 -> GreaterThanOrEqual16/2, GreaterThanOrEqual15/2
  Constant25/1 -> Equal11/2
  AND15/1 -> Receive Truck 3 Board 3 Calc Steering Angle/Enable
  Constant26/1 -> Receive Truck 3 Board 3 Calc Steering Angle/1(Input), Send can message4/1(Can_ID)
  Constant24/1 -> Equal12/2
  Data Store Read19/1 -> Equal14/1
  GreaterThanOrEqual17/1 -> AND17/1
  AND17/1 -> If Action Subsystem1/Enable
  Constant29/1 -> GreaterThanOrEqual17/2
  Constant30/1 -> Equal13/2
  Constant31/1 -> Equal14/2
  Data Store Read18/1 -> Equal13/1
  Equal14/1 -> AND17/3
  Equal13/1 -> AND17/2
  Data Store Read20/1 -> Equal15/1
  Equal16/1 -> AND18/3
  Equal15/1 -> AND18/2
  Constant32/1 -> Equal15/2
  Constant33/1 -> Equal16/2
  GreaterThanOrEqual18/1 -> AND18/1
  Data Store Read21/1 -> Equal16/1
  Constant34/1 -> GreaterThanOrEqual18/2
  AND18/1 -> If Action Subsystem2/Enable
  GreaterThanOrEqual19/1 -> If Action Subsystem3/Enable
  Data Type Conversion3/1 -> GreaterThanOrEqual8/1, GreaterThanOrEqual11/1, GreaterThanOrEqual3/1, GreaterThanOrEqual19/1, GreaterThanOrEqual18/1, GreaterThanOrEqual17/1, GreaterThanOrEqual14/1, GreaterThanOrEqual16/1, GreaterThanOrEqual15/1, GreaterThanOrEqual13/1, GreaterThanOrEqual2/1, GreaterThanOrEqual12/1, GreaterThanOrEqual10/1, GreaterThanOrEqual1/1, GreaterThanOrEqual9/1, GreaterThanOrEqual7/1, GreaterThanOrEqual6/1, GreaterThanOrEqual5/1, GreaterThanOrEqual4/1
  Constant37/1 -> GreaterThanOrEqual19/2
  Data Store Read10/1 -> Data Type Conversion2/1
  Data Type Conversion2/1 -> Send can message1/2(Can_Data)
  Data Type Conversion1/1 -> Send can message/2(Can_Data)
  Data Store Read4/1 -> Data Type Conversion1/1
  Data Type Conversion4/1 -> Send can message2/2(Can_Data)
  Data Store Read11/1 -> Data Type Conversion4/1
  Data Type Conversion5/1 -> Send can message3/2(Can_Data)
  Data Store Read12/1 -> Data Type Conversion5/1
  Data Type Conversion6/1 -> Send can message4/2(Can_Data)
  Data Store Read15/1 -> Data Type Conversion6/1

== system HANcoder_E407_DYS_MP/HANcoder STM32 Target - E407-STM32 algorithm/4.TTA Can System/4.3 TTA System/4.3.1 Initialization/Receive can message/CAN receive/Enabled Subsystem ==
  In1 : Inport
  In2 : Inport  Port=2
  In3 : Inport  Port=3
  In4 : Inport  Port=4
  In5 : Inport  Port=5
  In6 : Inport  Port=6
  In7 : Inport  Port=7
  In8 : Inport  Port=8
  Enable : EnablePort
  Out1 : Outport
  Out2 : Outport  Port=2
  Out3 : Outport  Port=3
  Out4 : Outport  Port=4
  Out5 : Outport  Port=5
  Out6 : Outport  Port=6
  Out7 : Outport  Port=7
  Out8 : Outport  Port=8
  wires:
  In8/1 -> Out8/1
  In7/1 -> Out7/1
  In6/1 -> Out6/1
  In5/1 -> Out5/1
  In4/1 -> Out4/1
  In3/1 -> Out3/1
  In2/1 -> Out2/1
  In1/1 -> Out1/1

== system HANcoder_E407_DYS_MP/HANcoder STM32 Target - E407-STM32 algorithm/4.TTA Can System/4.3 TTA System/4.3.1 Initialization/Receive can message/CAN receive2/Enabled Subsystem ==
  In1 : Inport
  In2 : Inport  Port=2
  In3 : Inport  Port=3
  In4 : Inport  Port=4
  In5 : Inport  Port=5
  In6 : Inport  Port=6
  In7 : Inport  Port=7
  In8 : Inport  Port=8
  Enable : EnablePort
  Out1 : Outport
  Out2 : Outport  Port=2
  Out3 : Outport  Port=3
  Out4 : Outport  Port=4
  Out5 : Outport  Port=5
  Out6 : Outport  Port=6
  Out7 : Outport  Port=7
  Out8 : Outport  Port=8
  wires:
  In8/1 -> Out8/1
  In7/1 -> Out7/1
  In6/1 -> Out6/1
  In5/1 -> Out5/1
  In4/1 -> Out4/1
  In3/1 -> Out3/1
  In2/1 -> Out2/1
  In1/1 -> Out1/1

== system HANcoder_E407_DYS_MP/HANcoder STM32 Target - E407-STM32 algorithm/4.TTA Can System/4.3 TTA System/4.3.3 Matrix Cycle Manager/4.3.3.1 Controller Matrix Cycle Truck Boards 1 2 and 3/4.3.3.1.1 controller basic cycle 0.1/Desync calculation ==
  note: Estimation of the Local Time when the message was sent
  note: Desync CAN1
      | expected RX - Actual RX
  note: Desync CAN2
      | expected RX - Actual RX
  TM_COMM : Inport
  New_msg_CAN1 : Inport  Port=2
  Enable : EnablePort  ShowOutputPort=on
  Constant : Constant  Commented=on  Value=COMM_Phase1
  Constant1 : Constant  Commented=on  Value=COMM_Phase2
  Constant2 : Constant  OutDataTypeStr=uint8
  Data Store Read1 : DataStoreRead  DataStoreName=Local_Ticks
  Data Store Read2 : DataStoreRead  DataStoreName=Local_Ticks
  Data Store Write1 : DataStoreWrite  Priority=23  DataStoreName=Desync_Ticks
  Data Store Write2 : DataStoreWrite  Priority=23  DataStoreName=SyncMesRec
  Minus : Sum  Priority=21  Inputs=+-
  Minus1 : Sum  Priority=20  Inputs=+-
  Sum : Sum  Priority=11  Inputs=+++
  Sum1 : Sum  Priority=13  Inputs=+++
  Switch1 : Switch  Priority=22  Criteria=u2 > Threshold
  delay_estimation_1 : Constant  Value=comm_delay_estimation1
  delay_estimation_2 : Constant  Value=comm_delay_estimation2
  wires:
  TM_COMM/1 -> Sum1/2, Sum/2
  delay_estimation_1/1 -> Sum/3
  delay_estimation_2/1 -> Sum1/3
  Constant1/1 -> Sum1/1
  Constant/1 -> Sum/1
  Minus1/1 -> Switch1/1
  Switch1/1 -> Data Store Write1/1  "DesyncTicks"
  New_msg_CAN1/1 -> Switch1/2
  Sum/1 -> Minus1/1  "EstimatedTimeCan1"
  Data Store Read2/1 -> Minus1/2  "LocalIncTicksMes"
  Data Store Read1/1 -> Minus/2  "LocalIncTicksMes2"
  Sum1/1 -> Minus/1  "EstimatedTimeCan2"
  Minus/1 -> Switch1/3
  Constant2/1 -> Data Store Write2/1

== system HANcoder_E407_DYS_MP/HANcoder STM32 Target - E407-STM32 algorithm/4.TTA Can System/4.3 TTA System/4.3.3 Matrix Cycle Manager/4.3.3.1 Controller Matrix Cycle Truck Boards 1 2 and 3/4.3.3.1.1 controller basic cycle 0.1/If Action Subsystem ==
  Enable : EnablePort  ShowOutputPort=on
  Constant1 : Constant  Value=2
  Constant2 : Constant  Value=0  OutDataTypeStr=uint8
  Counter1 : dspswit3/Counter  Direction=Up  CountEvent=Rising edge  CounterSize=User defined  MaxCount=255  InitialCount=0  Output=Count and Hit  HitValue=32  ResetInput=on  SamplesPerFrame=1  Ts=1  CntDtype=double  HitDtype=Logical
  Data Store Read : DataStoreRead  Priority=5  DataStoreName=Role_ID
  Data Store Read1 : DataStoreRead  DataStoreName=Desync_Ticks
  Data Store Read2 : DataStoreRead  DataStoreName=Local_Ticks
  Data Store Write1 : DataStoreWrite  Priority=23  DataStoreName=Local_Ticks
  Data Store Write2 : DataStoreWrite  Priority=23  DataStoreName=SyncMesRec
  Data Type Conversion : DataTypeConversion  OutDataTypeStr=uint16
  Equal : RelationalOperator  Operator===  OutDataTypeStr=boolean  RndMeth=Simplest
  Minus1 : Sum  Priority=20
  Switch1 : Switch  Priority=6  Criteria=u2 > Threshold
  Terminator1 : Terminator
  wires:
  Data Store Read1/1 -> Data Type Conversion/1
  Minus1/1 -> Switch1/1
  Data Type Conversion/1 -> Minus1/1
  Data Store Read/1 -> Equal/1
  Constant1/1 -> Equal/2
  Equal/1 -> Counter1/1, Switch1/2
  Switch1/1 -> Data Store Write1/1
  Data Store Read2/1 -> Switch1/3, Minus1/2
  Counter1/1 -> Terminator1/1  "ChancgeLocalTicks"
  Constant2/1 -> Data Store Write2/1

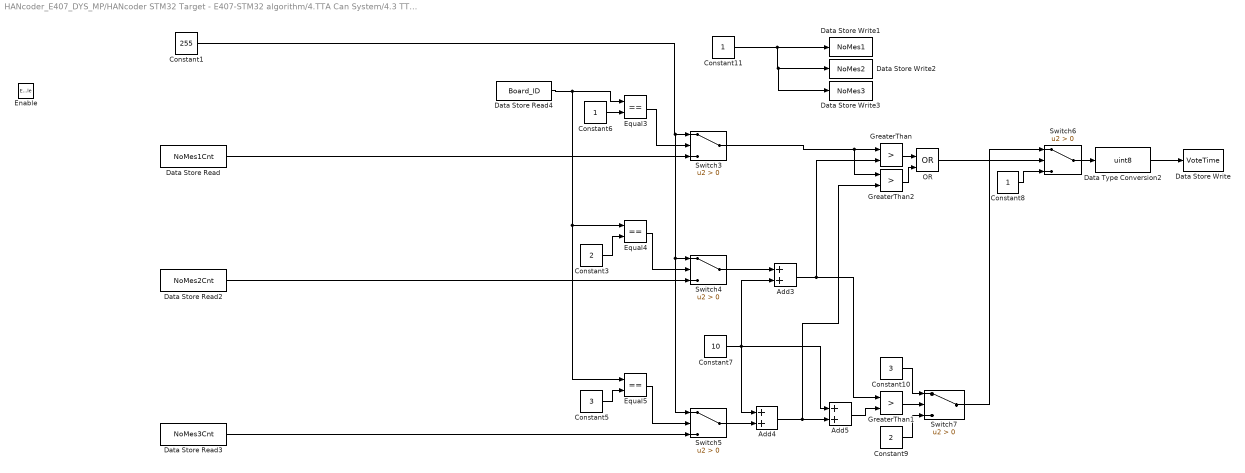
== system HANcoder_E407_DYS_MP/HANcoder STM32 Target - E407-STM32 algorithm/4.TTA Can System/4.3 TTA System/4.3.3 Matrix Cycle Manager/4.3.3.1 Controller Matrix Cycle Truck Boards 1 2 and 3/4.3.3.1.1 controller basic cycle 0.1/If Action Subsystem1 ==
  Enable : EnablePort  ShowOutputPort=on
  Add3 : Sum
  Add4 : Sum
  Add5 : Sum
  Constant1 : Constant  Value=255
  Constant10 : Constant  Value=3
  Constant11 : Constant
  Constant3 : Constant  Value=2
  Constant5 : Constant  Value=3
  Constant6 : Constant
  Constant7 : Constant  Value=10
  Constant8 : Constant
  Constant9 : Constant  Value=2
  Data Store Read : DataStoreRead  DataStoreName=NoMes1Cnt
  Data Store Read2 : DataStoreRead  DataStoreName=NoMes2Cnt
  Data Store Read3 : DataStoreRead  DataStoreName=NoMes3Cnt
  Data Store Read4 : DataStoreRead  DataStoreName=Board_ID
  Data Store Write : DataStoreWrite  DataStoreName=VoteTime
  Data Store Write1 : DataStoreWrite  DataStoreName=NoMes1
  Data Store Write2 : DataStoreWrite  DataStoreName=NoMes2
  Data Store Write3 : DataStoreWrite  DataStoreName=NoMes3
  Data Type Conversion2 : DataTypeConversion  OutDataTypeStr=uint8
  Equal3 : RelationalOperator  Operator===  OutDataTypeStr=boolean  RndMeth=Simplest
  Equal4 : RelationalOperator  Operator===  OutDataTypeStr=boolean  RndMeth=Simplest
  Equal5 : RelationalOperator  Operator===  OutDataTypeStr=boolean  RndMeth=Simplest
  GreaterThan : RelationalOperator  Operator=>  OutDataTypeStr=boolean  RndMeth=Simplest
  GreaterThan1 : RelationalOperator  Operator=>  OutDataTypeStr=boolean  RndMeth=Simplest
  GreaterThan2 : RelationalOperator  Operator=>  OutDataTypeStr=boolean  RndMeth=Simplest
  OR : Logic  Operator=OR  IconShape=distinctive  AllPortsSameDT=off  OutDataTypeStr=boolean
  Switch{3..7} (5 alike) : Switch  Criteria=u2 > Threshold
  wires:
  Constant6/1 -> Equal3/2
  Equal3/1 -> Switch3/2
  Data Store Read/1 -> Switch3/3
  Equal4/1 -> Switch4/2
  Data Store Read2/1 -> Switch4/3
  Constant3/1 -> Equal4/2
  Data Store Read4/1 -> Equal5/1, Equal4/1, Equal3/1
  Constant5/1 -> Equal5/2
  Equal5/1 -> Switch5/2
  Data Store Read3/1 -> Switch5/3
  Constant1/1 -> Switch5/1, Switch4/1, Switch3/1
  Switch4/1 -> Add3/1
  Switch5/1 -> Add4/2
  Constant7/1 -> Add5/1, Add3/2, Add4/1
  Switch3/1 -> GreaterThan2/1, GreaterThan/1
  Add3/1 -> GreaterThan/2, GreaterThan1/1
  Constant8/1 -> Switch6/3
  Switch7/1 -> Switch6/1
  Add4/1 -> GreaterThan2/2, Add5/2
  GreaterThan1/1 -> Switch7/2
  Add5/1 -> GreaterThan1/2
  GreaterThan/1 -> OR/1
  GreaterThan2/1 -> OR/2
  OR/1 -> Switch6/2
  Constant9/1 -> Switch7/3
  Constant10/1 -> Switch7/1
  Data Type Conversion2/1 -> Data Store Write/1
  Switch6/1 -> Data Type Conversion2/1
  Constant11/1 -> Data Store Write3/1, Data Store Write2/1, Data Store Write1/1

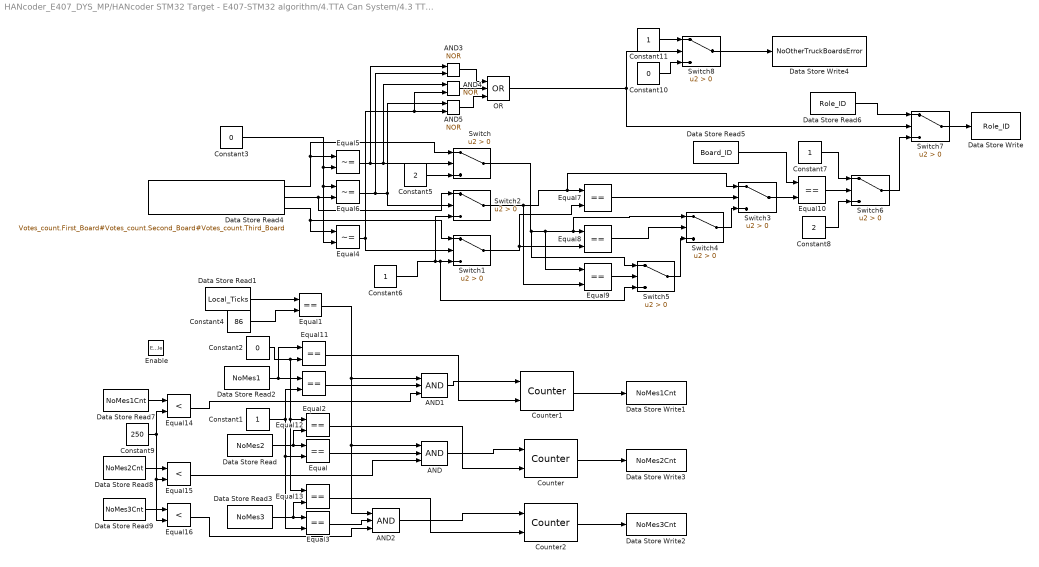
== system HANcoder_E407_DYS_MP/HANcoder STM32 Target - E407-STM32 algorithm/4.TTA Can System/4.3 TTA System/4.3.3 Matrix Cycle Manager/4.3.3.1 Controller Matrix Cycle Truck Boards 1 2 and 3/4.3.3.1.1 controller basic cycle 0.1/If Action Subsystem2 ==
  Enable : EnablePort  ShowOutputPort=on
  AND : Logic  Inputs=3  IconShape=distinctive  AllPortsSameDT=off  OutDataTypeStr=boolean
  AND1 : Logic  Inputs=3  IconShape=distinctive  AllPortsSameDT=off  OutDataTypeStr=boolean
  AND2 : Logic  Inputs=3  IconShape=distinctive  AllPortsSameDT=off  OutDataTypeStr=boolean
  AND3 : Logic  Operator=NOR  IconShape=distinctive  AllPortsSameDT=off  OutDataTypeStr=boolean
  AND4 : Logic  Operator=NOR  IconShape=distinctive  AllPortsSameDT=off  OutDataTypeStr=boolean
  AND5 : Logic  Operator=NOR  IconShape=distinctive  AllPortsSameDT=off  OutDataTypeStr=boolean
  Constant{1,6..7,11} (4 alike) : Constant
  Constant10 : Constant  Value=0
  Constant2 : Constant  Value=0
  Constant3 : Constant  Value=0
  Constant4 : Constant  Value=86
  Constant5 : Constant  Value=2
  Constant8 : Constant  Value=2
  Constant9 : Constant  Value=250
  Counter : dspswit3/Counter  Direction=Up  CountEvent=Rising edge  CounterSize=User defined  MaxCount=255  InitialCount=0  Output=Count  HitValue=32  ResetInput=on  SamplesPerFrame=1  Ts=1  CntDtype=double  HitDtype=Logical
  Counter1 : dspswit3/Counter  Direction=Up  CountEvent=Rising edge  CounterSize=User defined  MaxCount=255  InitialCount=0  Output=Count  HitValue=32  ResetInput=on  SamplesPerFrame=1  Ts=1  CntDtype=double  HitDtype=Logical
  Counter2 : dspswit3/Counter  Direction=Up  CountEvent=Rising edge  CounterSize=User defined  MaxCount=255  InitialCount=0  Output=Count  HitValue=32  ResetInput=on  SamplesPerFrame=1  Ts=1  CntDtype=double  HitDtype=Logical
  Data Store Read : DataStoreRead  DataStoreName=NoMes2
  Data Store Read1 : DataStoreRead  DataStoreName=Local_Ticks
  Data Store Read2 : DataStoreRead  DataStoreName=NoMes1
  Data Store Read3 : DataStoreRead  DataStoreName=NoMes3
  Data Store Read4 : DataStoreRead  DataStoreName=Votes_count  DataStoreElements=Votes_count.First_Board#Votes_count.Second_Board#Votes_count.Third_Board
  Data Store Read5 : DataStoreRead  DataStoreName=Board_ID
  Data Store Read6 : DataStoreRead  DataStoreName=Role_ID
  Data Store Read7 : DataStoreRead  DataStoreName=NoMes1Cnt
  Data Store Read8 : DataStoreRead  DataStoreName=NoMes2Cnt
  Data Store Read9 : DataStoreRead  DataStoreName=NoMes3Cnt
  Data Store Write : DataStoreWrite  DataStoreName=Role_ID
  Data Store Write1 : DataStoreWrite  Priority=23  DataStoreName=NoMes1Cnt
  Data Store Write2 : DataStoreWrite  Priority=23  DataStoreName=NoMes3Cnt
  Data Store Write3 : DataStoreWrite  Priority=23  DataStoreName=NoMes2Cnt
  Data Store Write4 : DataStoreWrite  DataStoreName=NoOtherTruckBoardsError
  Equal{,1..3,7..13} (11 alike) : RelationalOperator  Operator===  OutDataTypeStr=boolean  RndMeth=Simplest
  Equal14 : RelationalOperator  Operator=<  OutDataTypeStr=boolean  RndMeth=Simplest
  Equal15 : RelationalOperator  Operator=<  OutDataTypeStr=boolean  RndMeth=Simplest
  Equal16 : RelationalOperator  Operator=<  OutDataTypeStr=boolean  RndMeth=Simplest
  Equal4 : RelationalOperator  Operator=~=  OutDataTypeStr=boolean  RndMeth=Simplest
  Equal5 : RelationalOperator  Operator=~=  OutDataTypeStr=boolean  RndMeth=Simplest
  Equal6 : RelationalOperator  Operator=~=  OutDataTypeStr=boolean  RndMeth=Simplest
  OR : Logic  Operator=OR  Inputs=3  IconShape=distinctive  AllPortsSameDT=off  OutDataTypeStr=boolean
  Switch{,1..8} (9 alike) : Switch  Criteria=u2 > Threshold
  wires:
  Counter/1 -> Data Store Write3/1
  Data Store Read/1 -> Equal12/2, Equal/1
  Equal/1 -> AND/2
  Data Store Read1/1 -> Equal1/1
  Constant4/1 -> Equal1/2
  AND/1 -> Counter/1
  Counter1/1 -> Data Store Write1/1
  Equal2/1 -> AND1/2
  Data Store Read2/1 -> Equal11/1, Equal2/1
  AND1/1 -> Counter1/1
  Counter2/1 -> Data Store Write2/1
  Equal3/1 -> AND2/2
  Data Store Read3/1 -> Equal13/2, Equal3/1
  AND2/1 -> Counter2/1
  Equal1/1 -> AND1/1, AND2/1, AND/1
  Constant1/1 -> Equal2/2, Equal3/2, Equal/2
  Data Store Read4/3 -> Equal4/1, Switch1/1
  Data Store Read4/1 -> Switch/1, Equal5/1
  Data Store Read4/2 -> Switch2/1, Equal6/2
  Constant3/1 -> Equal6/1, Equal4/2, Equal5/2
  Equal5/1 -> AND3/1, AND4/1, Switch/2
  Constant5/1 -> Switch/3
  Constant6/1 -> Switch5/3, Switch1/3, Switch2/3
  Equal4/1 -> Switch1/2, AND5/2, AND4/2
  Equal6/1 -> AND3/2, Switch2/2, AND5/1
  Switch2/1 -> Equal9/2, Switch3/1, Equal7/1
  Switch1/1 -> Equal7/2, Equal8/2
  Equal7/1 -> Switch3/2
  Switch/1 -> Switch5/1, Equal9/1, Switch4/1, Equal8/1
  Switch4/1 -> Switch3/3
  Equal8/1 -> Switch4/2
  Equal9/1 -> Switch5/2
  Switch5/1 -> Switch4/3
  Switch3/1 -> Equal10/2
  Data Store Read5/1 -> Equal10/1
  Equal10/1 -> Switch6/2
  AND3/1 -> OR/1
  AND4/1 -> OR/2
  AND5/1 -> OR/3
  OR/1 -> Switch8/2, Switch7/2
  Switch6/1 -> Switch7/3
  Constant7/1 -> Switch6/1
  Constant8/1 -> Switch6/3
  Data Store Read6/1 -> Switch7/1
  Switch7/1 -> Data Store Write/1
  Constant2/1 -> Equal12/1, Equal13/1, Equal11/2
  Equal12/1 -> Counter/2
  Equal11/1 -> Counter1/2
  Equal13/1 -> Counter2/2
  Data Store Read7/1 -> Equal14/1
  Equal14/1 -> AND1/3
  Constant9/1 -> Equal16/2, Equal15/2, Equal14/2
  Equal15/1 -> AND/3
  Data Store Read8/1 -> Equal15/1
  Data Store Read9/1 -> Equal16/1
  Equal16/1 -> AND2/3
  Switch8/1 -> Data Store Write4/1
  Constant11/1 -> Switch8/1
  Constant10/1 -> Switch8/3
